simulink model "aa"  (R2019b)
settings: Solver=ode45  StartTime=0.0  StopTime=5  RelTol=1e-3  EnableMultiTasking=on
settings Model: Creator=casa  LastModifiedBy=bhisma
settings DataIOCC: LimitDataPoints=on  SaveFormat=Array  ReturnWorkspaceOutputs=off
settings OptimizationCC: LifeSpan=inf
settings DebuggingCC: SFUnexpectedBacktrackingDiag=warning  SFNoUnconditionalDefaultTransitionDiag=warning  SFExecutionAtInitializationDiag=none  ArithmeticOperatorsInVariantConditions=warning
settings HardwareCC: ProdBitPerPointer=32  ProdBitPerSizeT=32  ProdBitPerPtrDiffT=32  ProdLargestAtomicFloat=None  ProdIntDivRoundTo=Undefined  ProdEndianess=Unspecified  ProdWordSize=32  ProdHWDeviceType=32-bit Generic
settings ModelReferenceCC: PropagateSignalLabelsOutOfModel=off
settings SFSimCC: SimUseLocalCustomCode=off  CustomCodeUndefinedFunction=UseInterfaceOnly
settings RTWCC: RTWUseLocalCustomCode=off
settings CodeAppCC: StateflowObjectComments=on
settings GRTTargetCC: TargetLangStandard=C89/C90 (ANSI)  GeneratePreprocessorConditionals=Disable all
settings ConfigComp: CovMetricSettings=dw  CovHtmlReporting=on  CovSaveCumulativeToWorkspaceVar=on  CovSaveSingleToWorkspaceVar=on  CovExternalEMLEnable=off

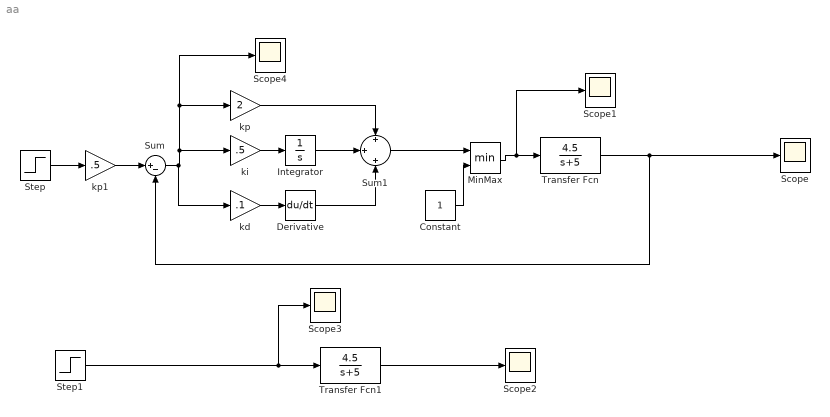
== system aa ==
  Constant : Constant
  Derivative : Derivative
  Integrator : Integrator
  MinMax : MinMax  Inputs=2
  Scope{,1..4} (5 alike) : Scope
  Step : Step  Time=0  SampleTime=0
  Step1 : Step  Time=0  SampleTime=0
  Sum : Sum  Inputs=|+-
  Sum1 : Sum  Inputs=+|+|+
  Transfer Fcn : TransferFcn  Numerator=[4.5]  Denominator=[1 5]
  Transfer Fcn1 : TransferFcn  Numerator=[4.5]  Denominator=[1 5]
  kd : Gain  Gain=.1
  ki : Gain  Gain=.5
  kp : Gain  Gain=2
  kp1 : Gain  Gain=.5
  wires:
  Sum/1 -> kd/1, ki/1, Scope4/1, kp/1
  Step1/1 -> Scope3/1, Transfer Fcn1/1
  Transfer Fcn1/1 -> Scope2/1
  Transfer Fcn/1 -> Scope/1, Sum/2
  MinMax/1 -> Scope1/1, Transfer Fcn/1
  Constant/1 -> MinMax/2
  Sum1/1 -> MinMax/1
  kp/1 -> Sum1/1
  kd/1 -> Derivative/1
  Derivative/1 -> Sum1/3
  ki/1 -> Integrator/1
  Integrator/1 -> Sum1/2
  Step/1 -> kp1/1
  kp1/1 -> Sum/1
